simulink model "Simulink"  (R2021b)
settings: Solver=VariableStepAuto  StartTime=0.0  StopTime=0.0001  RelTol=1e-3
libraries: dsparch4 x1
settings Model: Creator=Ehab Mansour  LastModifiedBy=ameir
settings SolverCC: AlgebraicLoopSolver=TrustRegion
settings DataIOCC: ReturnWorkspaceOutputs=off
settings DebuggingCC: SFMachineParentedDataDiag=warning  ArithmeticOperatorsInVariantConditions=warning
settings SFSimCC: SimUseLocalCustomCode=off  CustomCodeUndefinedFunction=UseInterfaceOnly
settings RTWCC: RTWUseLocalCustomCode=off

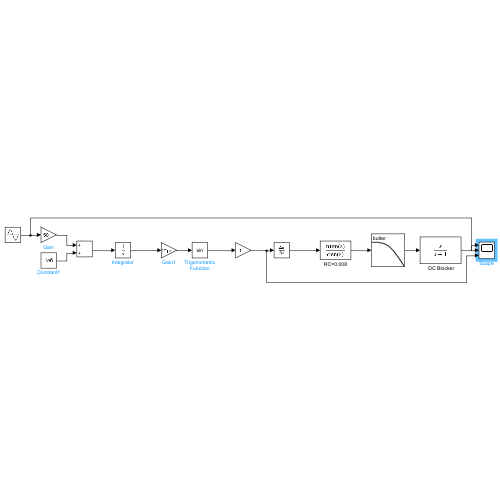
[thumbnail: Simulink's stored preview of the top-level diagram]
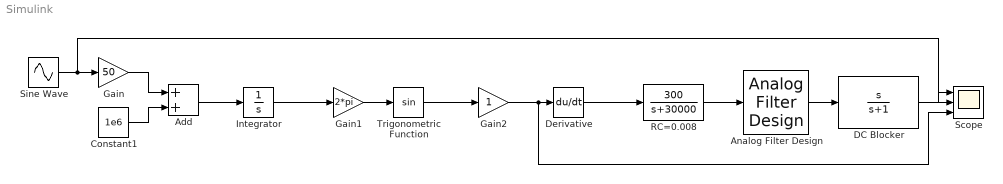
== system Simulink ==
  " DC Blocker" : TransferFcn  Numerator=[1 0]  Denominator=[1 1]
  Add : Sum
  Analog Filter Design : dsparch4/Analog Filter Design  method=Butterworth  filttype=Lowpass  N=1  Wlo=2*pi*10000  Whi=80  Rp=2  Rs=40
  Constant1 : Constant  Value=1e6
  Derivative : Derivative
  Gain : Gain  Gain=50
  Gain1 : Gain  Gain=2*pi
  Gain2 : Gain
  Integrator : Integrator
  "RC=0.008 " : TransferFcn  Numerator=[300]  Denominator=[1 30000]
  Scope : Scope  NumInputPorts=3
  Sine Wave : Sin  Amplitude=10  Frequency=2*pi*10000  SampleTime=0
  Trigonometric Function : Trigonometry
  wires:
  Sine Wave/1 -> Scope/2, Gain/1
  Gain/1 -> Add/1
  Constant1/1 -> Add/2
  Add/1 -> Integrator/1
  Integrator/1 -> Gain1/1
  Gain1/1 -> Trigonometric Function/1
  Trigonometric Function/1 -> Gain2/1
  Gain2/1 -> Scope/3, Derivative/1
  Analog Filter Design/1 -> " DC Blocker"/1
  "RC=0.008 "/1 -> Analog Filter Design/1
  Derivative/1 -> "RC=0.008 "/1
  " DC Blocker"/1 -> Scope/1
